simulink model "gm_soc_dvbs2_fpga"  (R2025b)
settings: Solver=VariableStepAuto  StartTime=0.0  StopTime=10.0  RelTol=1e-3
InitFcn:
  | soc_dvbs2_init;
undefined symbols (not defined in the file or in its folder): Add, coefficientsLog, coefficientsSqrt1, coefficientsSqrt2, dataBits, Deinterleaver, designMultirateFIR, noisePow, Shift, Short, soc_dvbs2_designFIRFilter, soc_dvbs2_txPacketBits, syncWord, txDataOut, txFiltCoeff, XData
libraries: simulink x304, hdlsllib x265, dspsigops x15, dsphdlfiltering2 x8, hdlmdlgenlib x6, dsphdlsigops2 x5, commseqgen3 x5, dsphdlmathfun2 x3, hwlogicconnlib x2, whdledac x2, commhdlcrc x2, whdlutilities x1
(part 17 of 36)

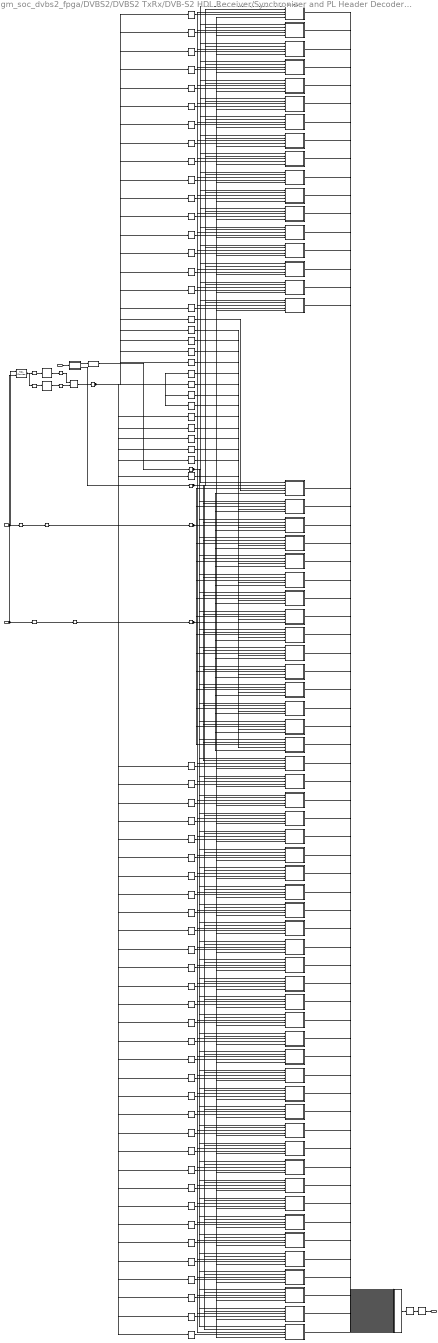
== system gm_soc_dvbs2_fpga/DVBS2/DVBS2 TxRx/DVB-S2 HDL Receiver/Synchronizer and PL Header Decoder/PL Header Recovery/PL Header Decoder/ML Decoder ==
  dataIn : Inport  OutDataTypeStr=fixdt(1, 18, 13)  PortDimensions=1  SampleTime=2.5e-07
  PLSCValid32 : Inport  Port=2  OutDataTypeStr=boolean  PortDimensions=1  SampleTime=2.5e-07
  reset : Inport  Port=3  OutDataTypeStr=boolean  PortDimensions=1  SampleTime=2.5e-07
  Code Word LUT 1 to 32 : LookupNDDirect  NumberOfTableDimensions=1  Table=config.intColAllCodeWords1to32
  Code Word LUT 33 to 64 : LookupNDDirect  NumberOfTableDimensions=1  Table=config.intColAllCodeWords33to64
  Compute Euclidean Distance : Subsystem
  Data Type Conversion1 : DataTypeConversion  OutDataTypeStr=fixdt(1,25,15)  SaturateOnIntegerOverflow=off  RndMeth=Floor
  Delay{1..2,9..14} (8 alike) : Delay
  Delay{15..19} (5 alike) : Delay  DelayLength=1
  Euclidean Distance Sum Up_instance1 : Subsystem
  Euclidean Distance Sum Up_instance10 : Subsystem
  Euclidean Distance Sum Up_instance11 : Subsystem
  Euclidean Distance Sum Up_instance12 : Subsystem
  Euclidean Distance Sum Up_instance13 : Subsystem
  Euclidean Distance Sum Up_instance14 : Subsystem
  Euclidean Distance Sum Up_instance15 : Subsystem
  Euclidean Distance Sum Up_instance16 : Subsystem
  Euclidean Distance Sum Up_instance17 : Subsystem
  Euclidean Distance Sum Up_instance18 : Subsystem
  Euclidean Distance Sum Up_instance19 : Subsystem
  Euclidean Distance Sum Up_instance2 : Subsystem
  Euclidean Distance Sum Up_instance20 : Subsystem
  Euclidean Distance Sum Up_instance21 : Subsystem
  Euclidean Distance Sum Up_instance22 : Subsystem
  Euclidean Distance Sum Up_instance23 : Subsystem
  Euclidean Distance Sum Up_instance24 : Subsystem
  Euclidean Distance Sum Up_instance25 : Subsystem
  Euclidean Distance Sum Up_instance26 : Subsystem
  Euclidean Distance Sum Up_instance27 : Subsystem
  Euclidean Distance Sum Up_instance28 : Subsystem
  Euclidean Distance Sum Up_instance29 : Subsystem
  Euclidean Distance Sum Up_instance3 : Subsystem
  Euclidean Distance Sum Up_instance30 : Subsystem
  Euclidean Distance Sum Up_instance31 : Subsystem
  Euclidean Distance Sum Up_instance32 : Subsystem
  Euclidean Distance Sum Up_instance33 : Subsystem
  Euclidean Distance Sum Up_instance34 : Subsystem
  Euclidean Distance Sum Up_instance35 : Subsystem
  Euclidean Distance Sum Up_instance36 : Subsystem
  Euclidean Distance Sum Up_instance37 : Subsystem
  Euclidean Distance Sum Up_instance38 : Subsystem
  Euclidean Distance Sum Up_instance39 : Subsystem
  Euclidean Distance Sum Up_instance4 : Subsystem
  Euclidean Distance Sum Up_instance40 : Subsystem
  Euclidean Distance Sum Up_instance41 : Subsystem
  Euclidean Distance Sum Up_instance42 : Subsystem
  Euclidean Distance Sum Up_instance43 : Subsystem
  Euclidean Distance Sum Up_instance44 : Subsystem
  Euclidean Distance Sum Up_instance45 : Subsystem
  Euclidean Distance Sum Up_instance46 : Subsystem
  Euclidean Distance Sum Up_instance47 : Subsystem
  Euclidean Distance Sum Up_instance48 : Subsystem
  Euclidean Distance Sum Up_instance49 : Subsystem
  Euclidean Distance Sum Up_instance5 : Subsystem
  Euclidean Distance Sum Up_instance50 : Subsystem
  Euclidean Distance Sum Up_instance51 : Subsystem
  Euclidean Distance Sum Up_instance52 : Subsystem
  Euclidean Distance Sum Up_instance53 : Subsystem
  Euclidean Distance Sum Up_instance54 : Subsystem
  Euclidean Distance Sum Up_instance55 : Subsystem
  Euclidean Distance Sum Up_instance56 : Subsystem
  Euclidean Distance Sum Up_instance57 : Subsystem
  Euclidean Distance Sum Up_instance58 : Subsystem
  Euclidean Distance Sum Up_instance59 : Subsystem
  Euclidean Distance Sum Up_instance6 : Subsystem
  Euclidean Distance Sum Up_instance60 : Subsystem
  Euclidean Distance Sum Up_instance61 : Subsystem
  Euclidean Distance Sum Up_instance62 : Subsystem
  Euclidean Distance Sum Up_instance63 : Subsystem
  Euclidean Distance Sum Up_instance64 : Subsystem
  Euclidean Distance Sum Up_instance7 : Subsystem
  Euclidean Distance Sum Up_instance8 : Subsystem
  Euclidean Distance Sum Up_instance9 : Subsystem
  Get Min Index : Subsystem
  HDL Counter : hdlsllib/Sources/HDL Counter  CountType=Count limited  CountInit=0  CountStep=1  CountMax=length(config.intColAllCodeWords1to32)-1  CountFromType=Initial value  CountFrom=0  CountResetPort=on  CountLoadPort=off  CountEnbPort=on  CountDirPort=off  CountHitOutputPort=off  CountDataType=Unsigned  CountWordLen=nextpow2(length(config.intColAllCodeWords1to32)-1)  CountFracLen=0  CountSampTime=1
  Integer to Bit Convertor : Subsystem
  Selector_1 : Selector  InputPortWidth=64  IndexOptions=Index vector (dialog)  Indices=double(1)  OutputSizes=1
  Selector_10 : Selector  InputPortWidth=64  IndexOptions=Index vector (dialog)  Indices=double(10)  OutputSizes=1
  Selector_11 : Selector  InputPortWidth=64  IndexOptions=Index vector (dialog)  Indices=double(11)  OutputSizes=1
  Selector_12 : Selector  InputPortWidth=64  IndexOptions=Index vector (dialog)  Indices=double(12)  OutputSizes=1
  Selector_13 : Selector  InputPortWidth=64  IndexOptions=Index vector (dialog)  Indices=double(13)  OutputSizes=1
  Selector_14 : Selector  InputPortWidth=64  IndexOptions=Index vector (dialog)  Indices=double(14)  OutputSizes=1
  Selector_15 : Selector  InputPortWidth=64  IndexOptions=Index vector (dialog)  Indices=double(15)  OutputSizes=1
  Selector_16 : Selector  InputPortWidth=64  IndexOptions=Index vector (dialog)  Indices=double(16)  OutputSizes=1
  Selector_17 : Selector  InputPortWidth=64  IndexOptions=Index vector (dialog)  Indices=double(17)  OutputSizes=1
  Selector_18 : Selector  InputPortWidth=64  IndexOptions=Index vector (dialog)  Indices=double(18)  OutputSizes=1
  Selector_19 : Selector  InputPortWidth=64  IndexOptions=Index vector (dialog)  Indices=double(19)  OutputSizes=1
  Selector_2 : Selector  InputPortWidth=64  IndexOptions=Index vector (dialog)  Indices=double(2)  OutputSizes=1
  Selector_20 : Selector  InputPortWidth=64  IndexOptions=Index vector (dialog)  Indices=double(20)  OutputSizes=1
  Selector_21 : Selector  InputPortWidth=64  IndexOptions=Index vector (dialog)  Indices=double(21)  OutputSizes=1
  Selector_22 : Selector  InputPortWidth=64  IndexOptions=Index vector (dialog)  Indices=double(22)  OutputSizes=1
  Selector_23 : Selector  InputPortWidth=64  IndexOptions=Index vector (dialog)  Indices=double(23)  OutputSizes=1
  Selector_24 : Selector  InputPortWidth=64  IndexOptions=Index vector (dialog)  Indices=double(24)  OutputSizes=1
  Selector_25 : Selector  InputPortWidth=64  IndexOptions=Index vector (dialog)  Indices=double(25)  OutputSizes=1
  Selector_26 : Selector  InputPortWidth=64  IndexOptions=Index vector (dialog)  Indices=double(26)  OutputSizes=1
  Selector_27 : Selector  InputPortWidth=64  IndexOptions=Index vector (dialog)  Indices=double(27)  OutputSizes=1
  Selector_28 : Selector  InputPortWidth=64  IndexOptions=Index vector (dialog)  Indices=double(28)  OutputSizes=1
  Selector_29 : Selector  InputPortWidth=64  IndexOptions=Index vector (dialog)  Indices=double(29)  OutputSizes=1
  Selector_3 : Selector  InputPortWidth=64  IndexOptions=Index vector (dialog)  Indices=double(3)  OutputSizes=1
  Selector_30 : Selector  InputPortWidth=64  IndexOptions=Index vector (dialog)  Indices=double(30)  OutputSizes=1
  Selector_31 : Selector  InputPortWidth=64  IndexOptions=Index vector (dialog)  Indices=double(31)  OutputSizes=1
  Selector_32 : Selector  InputPortWidth=64  IndexOptions=Index vector (dialog)  Indices=double(32)  OutputSizes=1
  Selector_33 : Selector  InputPortWidth=64  IndexOptions=Index vector (dialog)  Indices=double(33)  OutputSizes=1
  Selector_34 : Selector  InputPortWidth=64  IndexOptions=Index vector (dialog)  Indices=double(34)  OutputSizes=1
  Selector_35 : Selector  InputPortWidth=64  IndexOptions=Index vector (dialog)  Indices=double(35)  OutputSizes=1
  Selector_36 : Selector  InputPortWidth=64  IndexOptions=Index vector (dialog)  Indices=double(36)  OutputSizes=1
  Selector_37 : Selector  InputPortWidth=64  IndexOptions=Index vector (dialog)  Indices=double(37)  OutputSizes=1
  Selector_38 : Selector  InputPortWidth=64  IndexOptions=Index vector (dialog)  Indices=double(38)  OutputSizes=1
  Selector_39 : Selector  InputPortWidth=64  IndexOptions=Index vector (dialog)  Indices=double(39)  OutputSizes=1
  Selector_4 : Selector  InputPortWidth=64  IndexOptions=Index vector (dialog)  Indices=double(4)  OutputSizes=1
  Selector_40 : Selector  InputPortWidth=64  IndexOptions=Index vector (dialog)  Indices=double(40)  OutputSizes=1
  Selector_41 : Selector  InputPortWidth=64  IndexOptions=Index vector (dialog)  Indices=double(41)  OutputSizes=1
  Selector_42 : Selector  InputPortWidth=64  IndexOptions=Index vector (dialog)  Indices=double(42)  OutputSizes=1
  Selector_43 : Selector  InputPortWidth=64  IndexOptions=Index vector (dialog)  Indices=double(43)  OutputSizes=1
  Selector_44 : Selector  InputPortWidth=64  IndexOptions=Index vector (dialog)  Indices=double(44)  OutputSizes=1
  Selector_45 : Selector  InputPortWidth=64  IndexOptions=Index vector (dialog)  Indices=double(45)  OutputSizes=1
  Selector_46 : Selector  InputPortWidth=64  IndexOptions=Index vector (dialog)  Indices=double(46)  OutputSizes=1
  Selector_47 : Selector  InputPortWidth=64  IndexOptions=Index vector (dialog)  Indices=double(47)  OutputSizes=1
  Selector_48 : Selector  InputPortWidth=64  IndexOptions=Index vector (dialog)  Indices=double(48)  OutputSizes=1
  Selector_49 : Selector  InputPortWidth=64  IndexOptions=Index vector (dialog)  Indices=double(49)  OutputSizes=1
  Selector_5 : Selector  InputPortWidth=64  IndexOptions=Index vector (dialog)  Indices=double(5)  OutputSizes=1
  Selector_50 : Selector  InputPortWidth=64  IndexOptions=Index vector (dialog)  Indices=double(50)  OutputSizes=1
  Selector_51 : Selector  InputPortWidth=64  IndexOptions=Index vector (dialog)  Indices=double(51)  OutputSizes=1
  Selector_52 : Selector  InputPortWidth=64  IndexOptions=Index vector (dialog)  Indices=double(52)  OutputSizes=1
  Selector_53 : Selector  InputPortWidth=64  IndexOptions=Index vector (dialog)  Indices=double(53)  OutputSizes=1
  Selector_54 : Selector  InputPortWidth=64  IndexOptions=Index vector (dialog)  Indices=double(54)  OutputSizes=1
  Selector_55 : Selector  InputPortWidth=64  IndexOptions=Index vector (dialog)  Indices=double(55)  OutputSizes=1
  Selector_56 : Selector  InputPortWidth=64  IndexOptions=Index vector (dialog)  Indices=double(56)  OutputSizes=1
  Selector_57 : Selector  InputPortWidth=64  IndexOptions=Index vector (dialog)  Indices=double(57)  OutputSizes=1
  Selector_58 : Selector  InputPortWidth=64  IndexOptions=Index vector (dialog)  Indices=double(58)  OutputSizes=1
  Selector_59 : Selector  InputPortWidth=64  IndexOptions=Index vector (dialog)  Indices=double(59)  OutputSizes=1
  Selector_6 : Selector  InputPortWidth=64  IndexOptions=Index vector (dialog)  Indices=double(6)  OutputSizes=1
  Selector_60 : Selector  InputPortWidth=64  IndexOptions=Index vector (dialog)  Indices=double(60)  OutputSizes=1
  Selector_61 : Selector  InputPortWidth=64  IndexOptions=Index vector (dialog)  Indices=double(61)  OutputSizes=1
  Selector_62 : Selector  InputPortWidth=64  IndexOptions=Index vector (dialog)  Indices=double(62)  OutputSizes=1
  Selector_63 : Selector  InputPortWidth=64  IndexOptions=Index vector (dialog)  Indices=double(63)  OutputSizes=1
  Selector_64 : Selector  InputPortWidth=64  IndexOptions=Index vector (dialog)  Indices=double(64)  OutputSizes=1
  Selector_7 : Selector  InputPortWidth=64  IndexOptions=Index vector (dialog)  Indices=double(7)  OutputSizes=1
  Selector_8 : Selector  InputPortWidth=64  IndexOptions=Index vector (dialog)  Indices=double(8)  OutputSizes=1
  Selector_9 : Selector  InputPortWidth=64  IndexOptions=Index vector (dialog)  Indices=double(9)  OutputSizes=1
  concatenate : Concatenate  NumInputs=64
  t : Reshape
  bits6Out : Outport  SampleTime=2.5e-07
  wires:
  Euclidean Distance Sum Up_instance43/1(CwEdMetric) -> concatenate/43
  Euclidean Distance Sum Up_instance62/1(CwEdMetric) -> concatenate/62
  Get Min Index/1(out) -> bits6Out/1
  Euclidean Distance Sum Up_instance40/1(CwEdMetric) -> concatenate/40
  Euclidean Distance Sum Up_instance53/1(CwEdMetric) -> concatenate/53
  Selector_54/1 -> Euclidean Distance Sum Up_instance54/4(CWswitch)
  Selector_14/1 -> Euclidean Distance Sum Up_instance14/4(CWswitch)
  Delay16/1 -> Selector_64/1, Selector_61/1, Selector_59/1, Selector_57/1, Selector_54/1, Selector_53/1, Selector_52/1, Selector_46/1, Selector_45/1, Selector_44/1, Selector_41/1, Selector_40/1, Selector_36/1, Selector_33/1, Selector_32/1, Selector_28/1, Selector_27/1, Selector_26/1, Selector_25/1, Selector_23/1, Selector_22/1, Selector_21/1, Selector_20/1, Selector_18/1, Selector_15/1, Selector_12/1, Selector_11/1, Selector_9/1, Selector_7/1, Selector_6/1, Selector_5/1, Selector_4/1, Selector_3/1, Selector_16/1, Selector_13/1, Selector_60/1, Selector_1/1, Selector_38/1, Selector_62/1, Selector_34/1, Selector_8/1, Selector_58/1, Selector_56/1, Selector_43/1, Selector_10/1, Selector_63/1, Selector_14/1, Selector_31/1, Selector_55/1, Selector_35/1, Selector_30/1, Selector_2/1, Selector_29/1, Selector_47/1, Selector_19/1, Selector_39/1, Selector_49/1, Selector_42/1, Selector_24/1, Selector_50/1, Selector_17/1, Selector_51/1, Selector_48/1, Selector_37/1
  Euclidean Distance Sum Up_instance26/1(CwEdMetric) -> concatenate/26
  Euclidean Distance Sum Up_instance61/1(CwEdMetric) -> concatenate/61
  Selector_55/1 -> Euclidean Distance Sum Up_instance55/4(CWswitch)
  Euclidean Distance Sum Up_instance64/1(CwEdMetric) -> concatenate/64
  Euclidean Distance Sum Up_instance63/1(CwEdMetric) -> concatenate/63
  Euclidean Distance Sum Up_instance59/1(CwEdMetric) -> concatenate/59
  Euclidean Distance Sum Up_instance46/1(CwEdMetric) -> concatenate/46
  Selector_5/1 -> Euclidean Distance Sum Up_instance5/4(CWswitch)
  Selector_21/1 -> Euclidean Distance Sum Up_instance21/4(CWswitch)
  PLSCValid32/1 -> HDL Counter/2, Delay13/1
  Delay17/1 -> Euclidean Distance Sum Up_instance64/3(reset), Euclidean Distance Sum Up_instance63/3(reset), Euclidean Distance Sum Up_instance61/3(reset), Euclidean Distance Sum Up_instance57/3(reset), Euclidean Distance Sum Up_instance56/3(reset), Euclidean Distance Sum Up_instance55/3(reset), Euclidean Distance Sum Up_instance53/3(reset), Euclidean Distance Sum Up_instance52/3(reset), Euclidean Distance Sum Up_instance51/3(reset), Euclidean Distance Sum Up_instance50/3(reset), Euclidean Distance Sum Up_instance49/3(reset), Euclidean Distance Sum Up_instance48/3(reset), Euclidean Distance Sum Up_instance45/3(reset), Euclidean Distance Sum Up_instance43/3(reset), Euclidean Distance Sum Up_instance41/3(reset), Euclidean Distance Sum Up_instance37/3(reset), Euclidean Distance Sum Up_instance35/3(reset), Euclidean Distance Sum Up_instance33/3(reset), Euclidean Distance Sum Up_instance29/3(reset), Euclidean Distance Sum Up_instance23/3(reset), Euclidean Distance Sum Up_instance22/3(reset), Euclidean Distance Sum Up_instance21/3(reset), Euclidean Distance Sum Up_instance20/3(reset), Euclidean Distance Sum Up_instance32/3(reset), Euclidean Distance Sum Up_instance19/3(reset), Euclidean Distance Sum Up_instance17/3(reset), Euclidean Distance Sum Up_instance14/3(reset), Euclidean Distance Sum Up_instance13/3(reset), Euclidean Distance Sum Up_instance36/3(reset), Euclidean Distance Sum Up_instance12/3(reset), Euclidean Distance Sum Up_instance11/3(reset), Euclidean Distance Sum Up_instance10/3(reset), Euclidean Distance Sum Up_instance9/3(reset), Euclidean Distance Sum Up_instance8/3(reset), Euclidean Distance Sum Up_instance5/3(reset), Euclidean Distance Sum Up_instance24/3(reset), Euclidean Distance Sum Up_instance4/3(reset), Euclidean Distance Sum Up_instance62/3(reset), Euclidean Distance Sum Up_instance2/3(reset), Euclidean Distance Sum Up_instance59/3(reset), Euclidean Distance Sum Up_instance1/3(reset), Euclidean Distance Sum Up_instance38/3(reset), Euclidean Distance Sum Up_instance31/3(reset), Euclidean Distance Sum Up_instance44/3(reset), Euclidean Distance Sum Up_instance34/3(reset), Euclidean Distance Sum Up_instance18/3(reset), Euclidean Distance Sum Up_instance28/3(reset), Euclidean Distance Sum Up_instance46/3(reset), Euclidean Distance Sum Up_instance39/3(reset), Euclidean Distance Sum Up_instance58/3(reset), Euclidean Distance Sum Up_instance26/3(reset), Euclidean Distance Sum Up_instance40/3(reset), Euclidean Distance Sum Up_instance25/3(reset), Euclidean Distance Sum Up_instance6/3(reset), Euclidean Distance Sum Up_instance30/3(reset), Euclidean Distance Sum Up_instance47/3(reset), Euclidean Distance Sum Up_instance16/3(reset), Euclidean Distance Sum Up_instance27/3(reset), Euclidean Distance Sum Up_instance42/3(reset), Euclidean Distance Sum Up_instance3/3(reset), Euclidean Distance Sum Up_instance54/3(reset), Euclidean Distance Sum Up_instance15/3(reset), Euclidean Distance Sum Up_instance60/3(reset), Euclidean Distance Sum Up_instance7/3(reset)
  Delay19/1 -> Euclidean Distance Sum Up_instance62/1(Ed0), Euclidean Distance Sum Up_instance61/1(Ed0), Euclidean Distance Sum Up_instance60/1(Ed0), Euclidean Distance Sum Up_instance59/1(Ed0), Euclidean Distance Sum Up_instance58/1(Ed0), Euclidean Distance Sum Up_instance56/1(Ed0), Euclidean Distance Sum Up_instance54/1(Ed0), Euclidean Distance Sum Up_instance52/1(Ed0), Euclidean Distance Sum Up_instance50/1(Ed0), Euclidean Distance Sum Up_instance49/1(Ed0), Euclidean Distance Sum Up_instance48/1(Ed0), Euclidean Distance Sum Up_instance47/1(Ed0), Euclidean Distance Sum Up_instance45/1(Ed0), Euclidean Distance Sum Up_instance43/1(Ed0), Euclidean Distance Sum Up_instance42/1(Ed0), Euclidean Distance Sum Up_instance39/1(Ed0), Euclidean Distance Sum Up_instance37/1(Ed0), Euclidean Distance Sum Up_instance36/1(Ed0), Euclidean Distance Sum Up_instance35/1(Ed0), Euclidean Distance Sum Up_instance33/1(Ed0), Euclidean Distance Sum Up_instance46/1(Ed0), Euclidean Distance Sum Up_instance32/1(Ed0), Euclidean Distance Sum Up_instance31/1(Ed0), Euclidean Distance Sum Up_instance30/1(Ed0), Euclidean Distance Sum Up_instance29/1(Ed0), Euclidean Distance Sum Up_instance27/1(Ed0), Euclidean Distance Sum Up_instance26/1(Ed0), Euclidean Distance Sum Up_instance25/1(Ed0), Euclidean Distance Sum Up_instance53/1(Ed0), Euclidean Distance Sum Up_instance24/1(Ed0), Euclidean Distance Sum Up_instance23/1(Ed0), Euclidean Distance Sum Up_instance22/1(Ed0), Euclidean Distance Sum Up_instance21/1(Ed0), Euclidean Distance Sum Up_instance20/1(Ed0), Euclidean Distance Sum Up_instance19/1(Ed0), Euclidean Distance Sum Up_instance18/1(Ed0), Euclidean Distance Sum Up_instance17/1(Ed0), Euclidean Distance Sum Up_instance16/1(Ed0), Euclidean Distance Sum Up_instance15/1(Ed0), Euclidean Distance Sum Up_instance14/1(Ed0), Euclidean Distance Sum Up_instance13/1(Ed0), Euclidean Distance Sum Up_instance12/1(Ed0), Euclidean Distance Sum Up_instance11/1(Ed0), Euclidean Distance Sum Up_instance34/1(Ed0), Euclidean Distance Sum Up_instance8/1(Ed0), Euclidean Distance Sum Up_instance7/1(Ed0), Euclidean Distance Sum Up_instance6/1(Ed0), Euclidean Distance Sum Up_instance5/1(Ed0), Euclidean Distance Sum Up_instance4/1(Ed0), Euclidean Distance Sum Up_instance3/1(Ed0), Euclidean Distance Sum Up_instance2/1(Ed0), Euclidean Distance Sum Up_instance63/1(Ed0), Euclidean Distance Sum Up_instance40/1(Ed0), Euclidean Distance Sum Up_instance64/1(Ed0), Euclidean Distance Sum Up_instance41/1(Ed0), Euclidean Distance Sum Up_instance9/1(Ed0), Euclidean Distance Sum Up_instance28/1(Ed0), Euclidean Distance Sum Up_instance10/1(Ed0), Euclidean Distance Sum Up_instance51/1(Ed0), Euclidean Distance Sum Up_instance38/1(Ed0), Euclidean Distance Sum Up_instance1/1(Ed0), Euclidean Distance Sum Up_instance44/1(Ed0), Euclidean Distance Sum Up_instance57/1(Ed0), Euclidean Distance Sum Up_instance55/1(Ed0)
  Euclidean Distance Sum Up_instance58/1(CwEdMetric) -> concatenate/58
  Delay18/1 -> Euclidean Distance Sum Up_instance63/2(Ed1), Euclidean Distance Sum Up_instance59/2(Ed1), Euclidean Distance Sum Up_instance58/2(Ed1), Euclidean Distance Sum Up_instance55/2(Ed1), Euclidean Distance Sum Up_instance53/2(Ed1), Euclidean Distance Sum Up_instance52/2(Ed1), Euclidean Distance Sum Up_instance51/2(Ed1), Euclidean Distance Sum Up_instance49/2(Ed1), Euclidean Distance Sum Up_instance48/2(Ed1), Euclidean Distance Sum Up_instance46/2(Ed1), Euclidean Distance Sum Up_instance41/2(Ed1), Euclidean Distance Sum Up_instance40/2(Ed1), Euclidean Distance Sum Up_instance36/2(Ed1), Euclidean Distance Sum Up_instance35/2(Ed1), Euclidean Distance Sum Up_instance34/2(Ed1), Euclidean Distance Sum Up_instance32/2(Ed1), Euclidean Distance Sum Up_instance31/2(Ed1), Euclidean Distance Sum Up_instance28/2(Ed1), Euclidean Distance Sum Up_instance27/2(Ed1), Euclidean Distance Sum Up_instance26/2(Ed1), Euclidean Distance Sum Up_instance25/2(Ed1), Euclidean Distance Sum Up_instance24/2(Ed1), Euclidean Distance Sum Up_instance23/2(Ed1), Euclidean Distance Sum Up_instance22/2(Ed1), Euclidean Distance Sum Up_instance45/2(Ed1), Euclidean Distance Sum Up_instance21/2(Ed1), Euclidean Distance Sum Up_instance20/2(Ed1), Euclidean Distance Sum Up_instance19/2(Ed1), Euclidean Distance Sum Up_instance17/2(Ed1), Euclidean Distance Sum Up_instance15/2(Ed1), Euclidean Distance Sum Up_instance47/2(Ed1), Euclidean Distance Sum Up_instance10/2(Ed1), Euclidean Distance Sum Up_instance9/2(Ed1), Euclidean Distance Sum Up_instance7/2(Ed1), Euclidean Distance Sum Up_instance6/2(Ed1), Euclidean Distance Sum Up_instance3/2(Ed1), Euclidean Distance Sum Up_instance33/2(Ed1), Euclidean Distance Sum Up_instance62/2(Ed1), Euclidean Distance Sum Up_instance2/2(Ed1), Euclidean Distance Sum Up_instance1/2(Ed1), Euclidean Distance Sum Up_instance57/2(Ed1), Euclidean Distance Sum Up_instance12/2(Ed1), Euclidean Distance Sum Up_instance56/2(Ed1), Euclidean Distance Sum Up_instance30/2(Ed1), Euclidean Distance Sum Up_instance11/2(Ed1), Euclidean Distance Sum Up_instance5/2(Ed1), Euclidean Distance Sum Up_instance61/2(Ed1), Euclidean Distance Sum Up_instance64/2(Ed1), Euclidean Distance Sum Up_instance8/2(Ed1), Euclidean Distance Sum Up_instance37/2(Ed1), Euclidean Distance Sum Up_instance29/2(Ed1), Euclidean Distance Sum Up_instance14/2(Ed1), Euclidean Distance Sum Up_instance16/2(Ed1), Euclidean Distance Sum Up_instance50/2(Ed1), Euclidean Distance Sum Up_instance13/2(Ed1), Euclidean Distance Sum Up_instance39/2(Ed1), Euclidean Distance Sum Up_instance54/2(Ed1), Euclidean Distance Sum Up_instance43/2(Ed1), Euclidean Distance Sum Up_instance44/2(Ed1), Euclidean Distance Sum Up_instance18/2(Ed1), Euclidean Distance Sum Up_instance60/2(Ed1), Euclidean Distance Sum Up_instance4/2(Ed1), Euclidean Distance Sum Up_instance42/2(Ed1), Euclidean Distance Sum Up_instance38/2(Ed1)
  Euclidean Distance Sum Up_instance22/1(CwEdMetric) -> concatenate/22
  Euclidean Distance Sum Up_instance60/1(CwEdMetric) -> concatenate/60
  Euclidean Distance Sum Up_instance51/1(CwEdMetric) -> concatenate/51
  Euclidean Distance Sum Up_instance54/1(CwEdMetric) -> concatenate/54
  Euclidean Distance Sum Up_instance33/1(CwEdMetric) -> concatenate/33
  Delay1/1 -> Code Word LUT 33 to 64/1
  HDL Counter/1 -> Delay9/1, Delay1/1
  Euclidean Distance Sum Up_instance57/1(CwEdMetric) -> concatenate/57
  Euclidean Distance Sum Up_instance56/1(CwEdMetric) -> concatenate/56
  Euclidean Distance Sum Up_instance37/1(CwEdMetric) -> concatenate/37
  Selector_16/1 -> Euclidean Distance Sum Up_instance16/4(CWswitch)
  Euclidean Distance Sum Up_instance3/1(CwEdMetric) -> concatenate/3
  Euclidean Distance Sum Up_instance44/1(CwEdMetric) -> concatenate/44
  Euclidean Distance Sum Up_instance38/1(CwEdMetric) -> concatenate/38
  Euclidean Distance Sum Up_instance55/1(CwEdMetric) -> concatenate/55
  Euclidean Distance Sum Up_instance52/1(CwEdMetric) -> concatenate/52
  Euclidean Distance Sum Up_instance16/1(CwEdMetric) -> concatenate/16
  Euclidean Distance Sum Up_instance49/1(CwEdMetric) -> concatenate/49
  Selector_11/1 -> Euclidean Distance Sum Up_instance11/4(CWswitch)
  Delay15/1 -> Euclidean Distance Sum Up_instance64/5(validIn), Euclidean Distance Sum Up_instance63/5(validIn), Euclidean Distance Sum Up_instance61/5(validIn), Euclidean Distance Sum Up_instance60/5(validIn), Euclidean Distance Sum Up_instance56/5(validIn), Euclidean Distance Sum Up_instance54/5(validIn), Euclidean Distance Sum Up_instance53/5(validIn), Euclidean Distance Sum Up_instance50/5(validIn), Euclidean Distance Sum Up_instance48/5(validIn), Euclidean Distance Sum Up_instance39/5(validIn), Euclidean Distance Sum Up_instance40/5(validIn), Euclidean Distance Sum Up_instance35/5(validIn), Euclidean Distance Sum Up_instance33/5(validIn), Euclidean Distance Sum Up_instance30/5(validIn), Euclidean Distance Sum Up_instance29/5(validIn), Euclidean Distance Sum Up_instance26/5(validIn), Euclidean Distance Sum Up_instance25/5(validIn), Euclidean Distance Sum Up_instance24/5(validIn), Euclidean Distance Sum Up_instance23/5(validIn), Euclidean Distance Sum Up_instance21/5(validIn), Euclidean Distance Sum Up_instance19/5(validIn), Euclidean Distance Sum Up_instance18/5(validIn), Euclidean Distance Sum Up_instance13/5(validIn), Euclidean Distance Sum Up_instance42/5(validIn), Euclidean Distance Sum Up_instance8/5(validIn), Euclidean Distance Sum Up_instance5/5(validIn), Euclidean Distance Sum Up_instance4/5(validIn), Euclidean Distance Sum Up_instance3/5(validIn), Euclidean Distance Sum Up_instance2/5(validIn), Euclidean Distance Sum Up_instance6/5(validIn), Euclidean Distance Sum Up_instance15/5(validIn), Euclidean Distance Sum Up_instance51/5(validIn), Euclidean Distance Sum Up_instance58/5(validIn), Euclidean Distance Sum Up_instance47/5(validIn), Euclidean Distance Sum Up_instance44/5(validIn), Euclidean Distance Sum Up_instance10/5(validIn), Euclidean Distance Sum Up_instance37/5(validIn), Euclidean Distance Sum Up_instance34/5(validIn), Euclidean Distance Sum Up_instance1/5(validIn), Euclidean Distance Sum Up_instance43/5(validIn), Euclidean Distance Sum Up_instance59/5(validIn), Euclidean Distance Sum Up_instance22/5(validIn), Euclidean Distance Sum Up_instance17/5(validIn), Euclidean Distance Sum Up_instance27/5(validIn), Euclidean Distance Sum Up_instance62/5(validIn), Euclidean Distance Sum Up_instance31/5(validIn), Euclidean Distance Sum Up_instance57/5(validIn), Euclidean Distance Sum Up_instance9/5(validIn), Euclidean Distance Sum Up_instance12/5(validIn), Euclidean Distance Sum Up_instance38/5(validIn), Euclidean Distance Sum Up_instance49/5(validIn), Euclidean Distance Sum Up_instance14/5(validIn), Euclidean Distance Sum Up_instance20/5(validIn), Euclidean Distance Sum Up_instance41/5(validIn), Euclidean Distance Sum Up_instance16/5(validIn), Euclidean Distance Sum Up_instance36/5(validIn), Euclidean Distance Sum Up_instance28/5(validIn), Euclidean Distance Sum Up_instance45/5(validIn), Euclidean Distance Sum Up_instance11/5(validIn), Euclidean Distance Sum Up_instance32/5(validIn), Euclidean Distance Sum Up_instance7/5(validIn), Euclidean Distance Sum Up_instance46/5(validIn), Euclidean Distance Sum Up_instance52/5(validIn), Euclidean Distance Sum Up_instance55/5(validIn)
  Selector_40/1 -> Euclidean Distance Sum Up_instance40/4(CWswitch)
  Euclidean Distance Sum Up_instance50/1(CwEdMetric) -> concatenate/50
  Euclidean Distance Sum Up_instance41/1(CwEdMetric) -> concatenate/41
  Euclidean Distance Sum Up_instance25/1(CwEdMetric) -> concatenate/25
  Selector_22/1 -> Euclidean Distance Sum Up_instance22/4(CWswitch)
  Euclidean Distance Sum Up_instance35/1(CwEdMetric) -> concatenate/35
  Selector_39/1 -> Euclidean Distance Sum Up_instance39/4(CWswitch)
  Euclidean Distance Sum Up_instance42/1(CwEdMetric) -> concatenate/42
  Euclidean Distance Sum Up_instance36/1(CwEdMetric) -> concatenate/36
  Euclidean Distance Sum Up_instance48/1(CwEdMetric) -> concatenate/48
  Euclidean Distance Sum Up_instance12/1(CwEdMetric) -> concatenate/12
  Selector_36/1 -> Euclidean Distance Sum Up_instance36/4(CWswitch)
  Euclidean Distance Sum Up_instance47/1(CwEdMetric) -> concatenate/47
  Euclidean Distance Sum Up_instance7/1(CwEdMetric) -> concatenate/7
  Euclidean Distance Sum Up_instance45/1(CwEdMetric) -> concatenate/45
  Euclidean Distance Sum Up_instance13/1(CwEdMetric) -> concatenate/13
  Euclidean Distance Sum Up_instance39/1(CwEdMetric) -> concatenate/39
  Euclidean Distance Sum Up_instance8/1(CwEdMetric) -> concatenate/8
  Euclidean Distance Sum Up_instance29/1(CwEdMetric) -> concatenate/29
  Euclidean Distance Sum Up_instance21/1(CwEdMetric) -> concatenate/21
  Euclidean Distance Sum Up_instance34/1(CwEdMetric) -> concatenate/34
  Euclidean Distance Sum Up_instance27/1(CwEdMetric) -> concatenate/27
  Euclidean Distance Sum Up_instance24/1(CwEdMetric) -> concatenate/24
  Selector_1/1 -> Euclidean Distance Sum Up_instance1/4(CWswitch)
  Euclidean Distance Sum Up_instance2/1(CwEdMetric) -> concatenate/2
  Selector_2/1 -> Euclidean Distance Sum Up_instance2/4(CWswitch)
  Euclidean Distance Sum Up_instance32/1(CwEdMetric) -> concatenate/32
  Euclidean Distance Sum Up_instance31/1(CwEdMetric) -> concatenate/31
  Euclidean Distance Sum Up_instance30/1(CwEdMetric) -> concatenate/30
  Euclidean Distance Sum Up_instance28/1(CwEdMetric) -> concatenate/28
  Euclidean Distance Sum Up_instance23/1(CwEdMetric) -> concatenate/23
  Euclidean Distance Sum Up_instance20/1(CwEdMetric) -> concatenate/20
  Selector_56/1 -> Euclidean Distance Sum Up_instance56/4(CWswitch)
  Euclidean Distance Sum Up_instance19/1(CwEdMetric) -> concatenate/19
  Euclidean Distance Sum Up_instance14/1(CwEdMetric) -> concatenate/14
  Euclidean Distance Sum Up_instance18/1(CwEdMetric) -> concatenate/18
  Euclidean Distance Sum Up_instance17/1(CwEdMetric) -> concatenate/17
  Euclidean Distance Sum Up_instance15/1(CwEdMetric) -> concatenate/15
  Euclidean Distance Sum Up_instance9/1(CwEdMetric) -> concatenate/9
  Delay9/1 -> Code Word LUT 1 to 32/1
  Euclidean Distance Sum Up_instance5/1(CwEdMetric) -> concatenate/5
  Euclidean Distance Sum Up_instance11/1(CwEdMetric) -> concatenate/11
  Euclidean Distance Sum Up_instance10/1(CwEdMetric) -> concatenate/10
  Delay13/1 -> Delay14/1
  Euclidean Distance Sum Up_instance6/1(CwEdMetric) -> concatenate/6
  Euclidean Distance Sum Up_instance4/1(CwEdMetric) -> concatenate/4
  Euclidean Distance Sum Up_instance1/1(CwEdMetric) -> concatenate/1
  Selector_31/1 -> Euclidean Distance Sum Up_instance31/4(CWswitch)
  concatenate/1 -> t/1
  Selector_64/1 -> Euclidean Distance Sum Up_instance64/4(CWswitch)
  Selector_63/1 -> Euclidean Distance Sum Up_instance63/4(CWswitch)
  Selector_62/1 -> Euclidean Distance Sum Up_instance62/4(CWswitch)
  Selector_61/1 -> Euclidean Distance Sum Up_instance61/4(CWswitch)
  Selector_60/1 -> Euclidean Distance Sum Up_instance60/4(CWswitch)
  Selector_59/1 -> Euclidean Distance Sum Up_instance59/4(CWswitch)
  Compute Euclidean Distance/2(forBit1) -> Delay18/1
  Selector_58/1 -> Euclidean Distance Sum Up_instance58/4(CWswitch)
  t/1 -> Get Min Index/1(dataIn)
  Selector_57/1 -> Euclidean Distance Sum Up_instance57/4(CWswitch)
  Selector_53/1 -> Euclidean Distance Sum Up_instance53/4(CWswitch)
  Selector_52/1 -> Euclidean Distance Sum Up_instance52/4(CWswitch)
  Selector_51/1 -> Euclidean Distance Sum Up_instance51/4(CWswitch)
  Selector_50/1 -> Euclidean Distance Sum Up_instance50/4(CWswitch)
  Selector_49/1 -> Euclidean Distance Sum Up_instance49/4(CWswitch)
  Selector_48/1 -> Euclidean Distance Sum Up_instance48/4(CWswitch)
  Selector_34/1 -> Euclidean Distance Sum Up_instance34/4(CWswitch)
  Selector_47/1 -> Euclidean Distance Sum Up_instance47/4(CWswitch)
  Selector_46/1 -> Euclidean Distance Sum Up_instance46/4(CWswitch)
  Selector_45/1 -> Euclidean Distance Sum Up_instance45/4(CWswitch)
  Selector_44/1 -> Euclidean Distance Sum Up_instance44/4(CWswitch)
  Selector_43/1 -> Euclidean Distance Sum Up_instance43/4(CWswitch)
  Selector_42/1 -> Euclidean Distance Sum Up_instance42/4(CWswitch)
  Data Type Conversion1/1 -> Delay19/1
  Selector_41/1 -> Euclidean Distance Sum Up_instance41/4(CWswitch)
  Selector_38/1 -> Euclidean Distance Sum Up_instance38/4(CWswitch)
  Selector_37/1 -> Euclidean Distance Sum Up_instance37/4(CWswitch)
  Selector_35/1 -> Euclidean Distance Sum Up_instance35/4(CWswitch)
  Selector_33/1 -> Euclidean Distance Sum Up_instance33/4(CWswitch)
  Selector_32/1 -> Euclidean Distance Sum Up_instance32/4(CWswitch)
  Selector_30/1 -> Euclidean Distance Sum Up_instance30/4(CWswitch)
  Selector_29/1 -> Euclidean Distance Sum Up_instance29/4(CWswitch)
  Selector_28/1 -> Euclidean Distance Sum Up_instance28/4(CWswitch)
  Selector_27/1 -> Euclidean Distance Sum Up_instance27/4(CWswitch)
  Selector_26/1 -> Euclidean Distance Sum Up_instance26/4(CWswitch)
  Selector_25/1 -> Euclidean Distance Sum Up_instance25/4(CWswitch)
  Selector_24/1 -> Euclidean Distance Sum Up_instance24/4(CWswitch)
  Delay11/1 -> Delay12/1
  Selector_23/1 -> Euclidean Distance Sum Up_instance23/4(CWswitch)
  Selector_20/1 -> Euclidean Distance Sum Up_instance20/4(CWswitch)
  Selector_19/1 -> Euclidean Distance Sum Up_instance19/4(CWswitch)
  Delay2/1 -> Integer to Bit Convertor/2(LS)
  Selector_18/1 -> Euclidean Distance Sum Up_instance18/4(CWswitch)
  Selector_13/1 -> Euclidean Distance Sum Up_instance13/4(CWswitch)
  Selector_17/1 -> Euclidean Distance Sum Up_instance17/4(CWswitch)
  Selector_15/1 -> Euclidean Distance Sum Up_instance15/4(CWswitch)
  Selector_12/1 -> Euclidean Distance Sum Up_instance12/4(CWswitch)
  Delay12/1 -> Delay17/1
  Selector_10/1 -> Euclidean Distance Sum Up_instance10/4(CWswitch)
  Selector_9/1 -> Euclidean Distance Sum Up_instance9/4(CWswitch)
  Selector_8/1 -> Euclidean Distance Sum Up_instance8/4(CWswitch)
  Selector_7/1 -> Euclidean Distance Sum Up_instance7/4(CWswitch)
  Selector_6/1 -> Euclidean Distance Sum Up_instance6/4(CWswitch)
  Selector_4/1 -> Euclidean Distance Sum Up_instance4/4(CWswitch)
  Selector_3/1 -> Euclidean Distance Sum Up_instance3/4(CWswitch)
  Integer to Bit Convertor/1(Out1) -> Delay16/1
  Delay10/1 -> Integer to Bit Convertor/1(MS)
  Compute Euclidean Distance/1(forBit0) -> Data Type Conversion1/1
  Code Word LUT 33 to 64/1 -> Delay2/1
  Code Word LUT 1 to 32/1 -> Delay10/1
  dataIn/1 -> Compute Euclidean Distance/1(softBit)
  reset/1 -> Delay11/1, HDL Counter/1
  Delay14/1 -> Delay15/1

== system gm_soc_dvbs2_fpga/DVBS2/DVBS2 TxRx/DVB-S2 HDL Receiver/Synchronizer and PL Header Decoder/PL Header Recovery/PL Header Decoder/PLSC Descrambler ==
  dataIn : Inport  OutDataTypeStr=fixdt(1, 18, 13)  PortDimensions=1  SampleTime=2.5e-07
      settings: SignalType=complex
  resetIn : Inport  Port=2  OutDataTypeStr=boolean  PortDimensions=1  SampleTime=2.5e-07
  validIn : Inport  Port=3  OutDataTypeStr=boolean  PortDimensions=1  SampleTime=2.5e-07
  1-D Lookup Table : Lookup_n-D  NumberOfTableDimensions=1  LookupTableObject=''  BreakpointsSpecification=Even spacing  BreakpointsForDimension1=[-5:5]  BreakpointsForDimension1FirstPoint=0  BreakpointsForDimension2FirstPoint=10  BreakpointsForDimension2Spacing=12  IndexSearchMethod=Evenly spaced points  Table=config.PLSCDescramLUT  TableDataTypeStr=Inherit: Inherit from 'Table data'  InterpMethod=Flat  InternalRulePriority=Speed  OutDataTypeStr=fixdt(1, 2, 0)  RndMeth=Simplest
  Data Type Conversion : DataTypeConversion  OutDataTypeStr=boolean  SampleTime=2.5e-07  SaturateOnIntegerOverflow=off  RndMeth=Floor
  Delay{1..8} (8 alike) : Delay  DelayLength=double(1)  InitialCondition=0  SampleTime=2.5e-07
  Delay{9..27} (19 alike) : Delay  DelayLength=double(2)  InitialCondition=0  SampleTime=2.5e-07
  Math Function : Math  Operator=conj  OutDataTypeStr=fixdt(1, 2, 0)
  PLSC Valid Counter : hdlsllib/Sources/HDL Counter  CountType=Count limited  CountInit=0  CountStep=1  CountMax=length(config.PLSCDescramLUT)-1  CountFromType=Initial value  CountFrom=0  CountResetPort=on  CountLoadPort=off  CountEnbPort=on  CountDirPort=off  CountHitOutputPort=off  CountDataType=Unsigned  CountWordLen=nextpow2(length(config.PLSCDescramLUT)-1)  CountFracLen=0  CountSampTime=1
  Product : Product  Inputs=**  OutDataTypeStr=fixdt(1, 18, 13)  SampleTime=2.5e-07
  dtc1_Extract Bits : DataTypeConversion  OutDataTypeStr=fixdt(0, 1, 0)  SampleTime=2.5e-07  SaturateOnIntegerOverflow=off  RndMeth=Floor
  dataOut : Outport  SampleTime=2.5e-07
  indexIndicator : Outport  Port=2  SampleTime=2.5e-07
  validOut : Outport  Port=3  SampleTime=2.5e-07
  resetOut : Outport  Port=4  SampleTime=2.5e-07
  wires:
  resetIn/1 -> Delay1/1
  validIn/1 -> Delay2/1
  Delay1/1 -> Delay4/1, PLSC Valid Counter/1
  Delay4/1 -> Delay14/1
  Delay14/1 -> Delay18/1
  Delay2/1 -> Delay5/1, PLSC Valid Counter/2
  Delay22/1 -> Data Type Conversion/1
  Delay5/1 -> Delay13/1
  PLSC Valid Counter/1 -> Delay7/1, Delay6/1
  dataIn/1 -> Delay3/1
  Delay3/1 -> Delay8/1
  Delay13/1 -> Delay17/1
  Delay7/1 -> Delay9/1
  1-D Lookup Table/1 -> Delay10/1
  Delay6/1 -> Delay12/1
  Delay18/1 -> Delay24/1
  Delay17/1 -> Delay23/1
  Delay9/1 -> 1-D Lookup Table/1
  Delay27/1 -> resetOut/1
  Delay12/1 -> dtc1_Extract Bits/1
  Delay24/1 -> Delay27/1
  Delay8/1 -> Delay11/1
  Delay23/1 -> Delay26/1
  dtc1_Extract Bits/1 -> Delay16/1
  Delay26/1 -> validOut/1
  Delay11/1 -> Delay15/1
  Delay25/1 -> indexIndicator/1
  Delay10/1 -> Math Function/1
  Delay16/1 -> Delay22/1
  Delay15/1 -> Delay20/1
  Math Function/1 -> Delay19/1
  Delay20/1 -> Product/1
  Delay19/1 -> Product/2
  Data Type Conversion/1 -> Delay25/1
  Product/1 -> Delay21/1
  Delay21/1 -> dataOut/1

== system gm_soc_dvbs2_fpga/DVBS2/DVBS2 TxRx/DVB-S2 HDL Receiver/Synchronizer and PL Header Decoder/PL Header Recovery/PL Header Decoder/pi//2 BPSK Soft Bit Generator ==
  dataIn : Inport  OutDataTypeStr=fixdt(1, 18, 13)  PortDimensions=1  SampleTime=2.5e-07
      settings: SignalType=complex
  indexIndicatorIn : Inport  Port=2  OutDataTypeStr=boolean  PortDimensions=1  SampleTime=2.5e-07
  validIn : Inport  Port=3  OutDataTypeStr=boolean  PortDimensions=1  SampleTime=2.5e-07
  resetIn : Inport  Port=4  OutDataTypeStr=boolean  PortDimensions=1  SampleTime=2.5e-07
  Complex to Real-Imag : ComplexToRealImag  Output=Real
  Delay{1..12} (12 alike) : Delay
  Gain : Gain  Gain=fi(exp(1i*(3*pi/4)),1,16)  ParamDataTypeStr=Inherit: Inherit from 'Gain'  OutDataTypeStr=fixdt(1, 18, 13)
  Gain1 : Gain  Gain=fi(exp(1i*(pi/4)),1,16)  ParamDataTypeStr=Inherit: Inherit from 'Gain'  OutDataTypeStr=fixdt(1, 18, 13)
  Switch : Switch  Criteria=u2 ~= 0  OutDataTypeStr=fixdt(1, 18, 13)  SaturateOnIntegerOverflow=off  InputSameDT=off
  dataOut : Outport  SampleTime=2.5e-07
  indexIndicatorOut : Outport  Port=2  SampleTime=2.5e-07
  validOut : Outport  Port=3  SampleTime=2.5e-07
  resetOut : Outport  Port=4  SampleTime=2.5e-07
  wires:
  Switch/1 -> Complex to Real-Imag/1
  Delay3/1 -> Gain1/1
  Delay10/1 -> Delay12/1
  Delay9/1 -> Delay11/1
  dataIn/1 -> Delay3/1, Delay1/1
  validIn/1 -> Delay9/1
  Delay1/1 -> Gain/1
  Complex to Real-Imag/1 -> dataOut/1
  indexIndicatorIn/1 -> Delay7/1, Delay5/1
  Gain/1 -> Delay4/1
  resetIn/1 -> Delay10/1
  Delay8/1 -> indexIndicatorOut/1
  Delay11/1 -> validOut/1
  Gain1/1 -> Delay2/1
  Delay12/1 -> resetOut/1
  Delay5/1 -> Delay6/1
  Delay7/1 -> Delay8/1
  Delay6/1 -> Switch/2
  Delay2/1 -> Switch/1
  Delay4/1 -> Switch/3
